simulink model "Problem1"  (R2021a)
settings: Solver=ode45  StartTime=0.0  StopTime=10.0  RelTol=1e-3
values from neighbouring files (symbols this model uses):
  mu = 4    [Demo_4481.m]    (also in Homework1.m = 1)
  x_0 = 2    [Homework1.m]
  x_dot_0 = 2    [Homework1.m]
undefined symbols (not defined in the file or in its folder): DiscIntNeverNeededParam
settings Model: Creator=Willi  LastModifiedBy=Willi

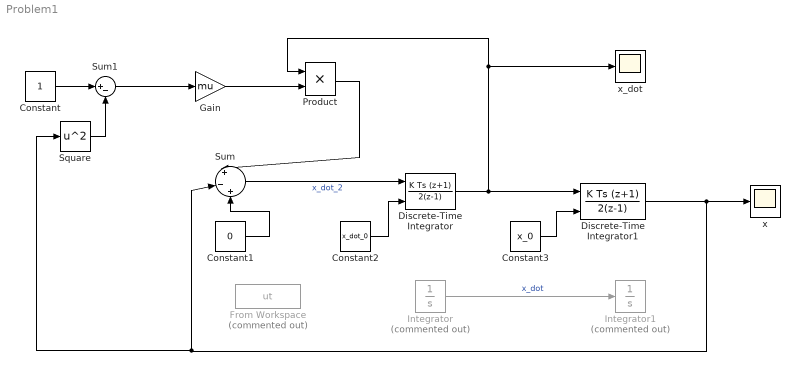
== system Problem1 ==
  Constant : Constant
  Constant1 : Constant  Value=0
  Constant2 : Constant  Value=x_dot_0
  Constant3 : Constant  Value=x_0
  Discrete-Time Integrator : DiscreteIntegrator  IntegratorMethod=Integration: Trapezoidal  InitialConditionSource=external  SampleTime=-1  ICPrevOutput=DiscIntNeverNeededParam  ICPrevScaledInput=DiscIntNeverNeededParam
  Discrete-Time Integrator1 : DiscreteIntegrator  IntegratorMethod=Integration: Trapezoidal  InitialConditionSource=external  SampleTime=-1  ICPrevOutput=DiscIntNeverNeededParam  ICPrevScaledInput=DiscIntNeverNeededParam
  From Workspace : FromWorkspace  Commented=on  VariableName=ut
  Gain : Gain  Gain=mu
  Integrator : Integrator  Commented=on  InitialCondition=2
  Integrator1 : Integrator  Commented=on  InitialCondition=2
  Product : Product
  Square : Math  Operator=square  SaturateOnIntegerOverflow=on
  Sum : Sum  Inputs=|+|-|+
  Sum1 : Sum  Inputs=|+-
  x : Scope
  x_dot : Scope
  wires:
  Sum/1 -> Discrete-Time Integrator/1  "x_dot_2"
  Integrator/1 -> Integrator1/1  "x_dot"
  Constant/1 -> Sum1/1
  Square/1 -> Sum1/2
  Sum1/1 -> Gain/1
  Gain/1 -> Product/2
  Product/1 -> Sum/1
  Constant1/1 -> Sum/3
  Discrete-Time Integrator/1 -> x_dot/1, Product/1, Discrete-Time Integrator1/1
  Discrete-Time Integrator1/1 -> x/1, Square/1, Sum/2
  Constant2/1 -> Discrete-Time Integrator/2
  Constant3/1 -> Discrete-Time Integrator1/2
